simulink library "Lib_EthernetCommunication"  (R2019b)
settings: Solver=VariableStepAuto  StartTime=0.0  StopTime=10.0  RelTol=1e-3
PostLoadFcn:
  | , if any(exist('dsrtsu_mdlpostloadfcn', 'file') == [2, 3, 6]), try dsrtsu_mdlpostloadfcn('Execute', bdroot); catch fprintf('Error in PostLoadFcn (dsrtsu_mdlpostloadfcn) for model "%s":\n %s\n', bdroot, lasterr); end, end,
undefined symbols (not defined in the file): a, acceleration, brake, ddkappa, default_control_command_apollo_bus, default_localization_bus, default_trajectory_bus, dkappa, kappa, n_trajectory_point, relative_time, s, sequence_num, steering_rate, steering_target, theta, throttle, timestamp_sec, v, x, y, z
libraries: rtiethernetudplib x4
settings Model: DSRTSU_INTERNAL_RTI_VER=550  DSRTSU_INTERNAL_RTI_TYPE=rti1401  RTICANMMDATA=struct('GeneralSetupData',struct('modelroot','C:\fav\stack\src\autobox\Simulink\Models','generalsettings',struct('filesettings',struct('destfolder',struct('Name','RTICANMM_FILES','Check',1),'buildfolder',struct('Name','.','Check',1),'AbsDestfolder',struct('Name','C:\fav\stack\src\autobox\Simulink\Models\RTICANMM_FILES'),'AbsBuildfolder',struct('Name','C:\fav\stack\src\autobox\Simulink\Models'))),'options',struct('addpaths',1,'rmpaths',1,'addtrcexclusion',logical(1),'cannavigator',struct('checkmonitoring',0),'show_usrtrc',0,'use_usrtrc',0),'advanced',struct('options',[1 1 1 1 1 1 1 1 1 1 1 1 1 1 1 1 1 1 1 1 1 1 1 1 1 1 1 1 1 1 1 1 1 1 1 1 1 1 1 1 1 1 1 1 1 1 1 1 1 1 1 1 1 1 1 1 1 1 1 1 1 1 1 1 1 1 1 1 1 1 1 1 1 1 1 1 1 1 1 1 1 1 1 1 1 1 1 1 1 1 1 1 1 1 1 1 1 1 1 1]),'MPSetup',{{}},'modelname','Lib_EthernetCommunication','block','Lib_EthernetCommunication'))  DSRTSU_INTERNAL_RTIFPGA=150  Creator=esterle  LastModifiedBy=kessler
settings DataIOCC: ReturnWorkspaceOutputs=off
settings DebuggingCC: ArithmeticOperatorsInVariantConditions=warning
settings SFSimCC: SimUseLocalCustomCode=off  CustomCodeUndefinedFunction=UseInterfaceOnly
settings RTWCC: RTWUseLocalCustomCode=off

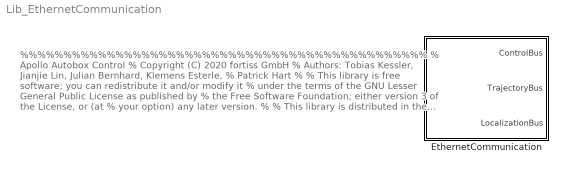
== system Lib_EthernetCommunication ==
  note: %%%%%%%%%%%%%%%%%%%%%%%%%%%%%%%%%%%%%%%%%%%%%%%
      | % Apollo Autobox Control
      | % Copyright (C) 2020 fortiss GmbH
      | % Authors: Tobias Kessler, Jianjie Lin, Julian Bernhard, Klemens Esterle,
      | % Patrick Hart
      | %
      | % This library is free software; you can redistribute it and/or modify it
      | % under the terms of the GNU Lesser General Public License as published by
      | % the Free Software Foundation; either version 3 of the License, or (at
      | % your option) any later version.
      | %
      | % This library is distributed in the hope that it will be useful, but
      | % WITHOUT ANY WARRANTY; without even the implied warranty of
      | % MERCHANTABILITY or FITNESS FOR A PARTICULAR PURPOSE. See the GNU Lesser
      | % General Public License for more details.
      | %
      | % You should have received a copy of the GNU Lesser General Public License
      | % along with this library; if not, write to the Free Software Foundation,
      | % Inc., 51 Franklin Street, Fifth Floor, Boston, MA 02110-1301, USA.
      | %%%%%%%%%%%%%%%%%%%%%%%%%%%%%%%%%%%%%%%%%%%%%%%
  EthernetCommunication : Subsystem

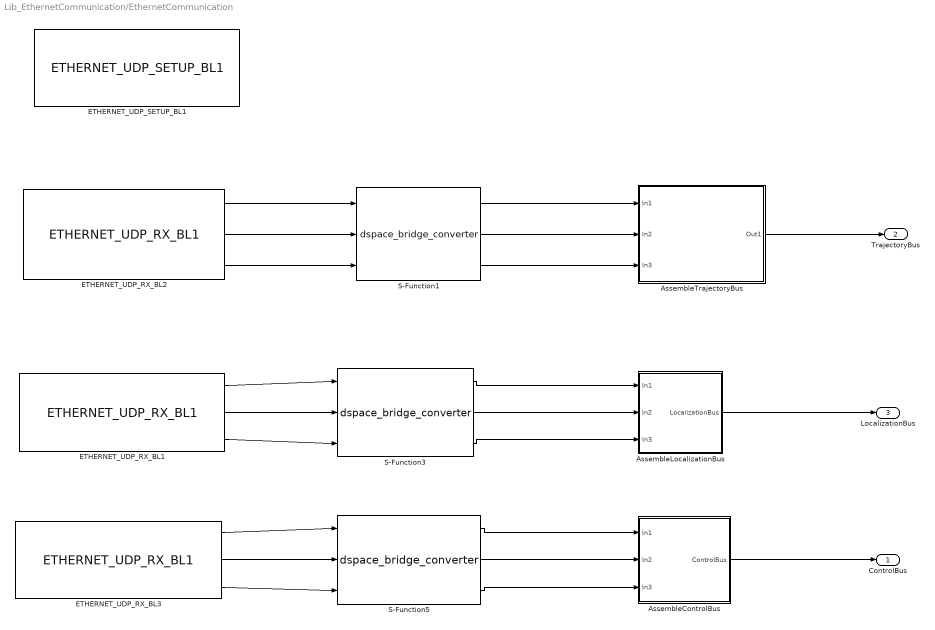
== system Lib_EthernetCommunication/EthernetCommunication ==
  AssembleControlBus : Subsystem
  AssembleLocalizationBus : Subsystem
  AssembleTrajectoryBus : Subsystem
  ETHERNET_UDP_RX_BL1 : rtiethernetudplib/ETHERNET_UDP_RX_BL1  InterfaceName=rti_ethernet_interface_name  BoardType=ETH Type 1  ModuleNo=1  ChannelNo=1  SocketNo=2  MaxMessageSize=1208  LocalSocket=192.168.140.1:5001  RemoteSocket=0.0.0.0:0  DSProperties=struct('RTI',struct('Version',uint32(1),'BlockType',struct('isSLSource',uint8(1),'isSLSink',uint8(0),'isHWSource',uint8(0),'isHWSink',uint8(1),'isSetup',uint8(0),'isInline',uint8(1),'isNonInline',uint8(1),'isInterrupt',uint8(0),'isChannelwise',uint8(1)),'IOBoardType','DSETHERNETUDP','UnitType','ETHUDP','Identifier','RX','DialogType','SL','BlockSet','RTIETHERNETUDP','SlaveProcessor','NONE'))  RTIBlockInterface=struct('OutputPortsWidth',int32([1 1 1]),'OutputPortsActive',[1 1 1],'OutputPortsName',{{'Data',['Message Size'],'Status'}},'OutputPortsDataType',{{'SS_UINT32','SS_INT32','SS_BOOLEAN'}},'BlockDisplay',{{['Ethernet UDP Receive\nBoard Type: ETH Type 1\nModule: 1\nSocket: 2\nMaximum Message Size: 1208'],'center'}},'IconTransparency','on','InitLevel',3,'BlockName',struct('Token',{{'ETHERNET_UDP_RX_BL1'}}),'MaskDescription',['To receive messages from the Ethernet UDP interface.'])  RTIBlockParameters=struct('InterfaceName',{{'rti_ethernet_interface_name','OFF',[]}},'BoardType',{{1,'OFF',[]}},'ModuleNo',{{1,'OFF',[1 16]}},'ChannelNo',{{1,'OFF',[1 2]}},'SocketNo',{{2,'OFF',[1 4]}},'MaxMessageSize',{{1208,'ON',[1 1472]}},'LocalSocket',{{'192.168.140.1:5001','OFF',[]}},'RemoteSocket',{{'0.0.0.0:0','OFF',[]}})  RTISFcnParameters=struct('InterfaceName','char','BoardType','double','ModuleNo','double','ChannelNo','double','SocketNo','double','MaxMessageSize','double','LocalSocket','char','RemoteSocket','char')  RTIBlockParaDefault=struct('InterfaceName','rti_ethernet_interface_name','BoardType',1,'ModuleNo',1,'ChannelNo',1,'SocketNo',1,'MaxMessageSize',625,'LocalSocket','XXX.XXX.XXX.XXX:5000','RemoteSocket','XXX.XXX.XXX.XXX:5000')
      settings: SourceProductName=dSPACE RTI Ethernet (UDP) Blockset
  ETHERNET_UDP_RX_BL2 : rtiethernetudplib/ETHERNET_UDP_RX_BL1  InterfaceName=rti_ethernet_interface_name  BoardType=ETH Type 1  ModuleNo=1  ChannelNo=1  SocketNo=1  MaxMessageSize=1208  LocalSocket=192.168.140.1:5000  RemoteSocket=0.0.0.0:0  DSProperties=struct('RTI',struct('Version',uint32(1),'BlockType',struct('isSLSource',uint8(1),'isSLSink',uint8(0),'isHWSource',uint8(0),'isHWSink',uint8(1),'isSetup',uint8(0),'isInline',uint8(1),'isNonInline',uint8(1),'isInterrupt',uint8(0),'isChannelwise',uint8(1)),'IOBoardType','DSETHERNETUDP','UnitType','ETHUDP','Identifier','RX','DialogType','SL','BlockSet','RTIETHERNETUDP','SlaveProcessor','NONE'))  RTIBlockInterface=struct('OutputPortsWidth',int32([1 1 1]),'OutputPortsActive',[1 1 1],'OutputPortsName',{{'Data',['Message Size'],'Status'}},'OutputPortsDataType',{{'SS_UINT32','SS_INT32','SS_BOOLEAN'}},'BlockDisplay',{{['Ethernet UDP Receive\nBoard Type: ETH Type 1\nModule: 1\nSocket: 1\nMaximum Message Size: 1208'],'center'}},'IconTransparency','on','InitLevel',3,'BlockName',struct('Token',{{'ETHERNET_UDP_RX_BL1'}}),'MaskDescription',['To receive messages from the Ethernet UDP interface.'])  RTIBlockParameters=struct('InterfaceName',{{'rti_ethernet_interface_name','OFF',[]}},'BoardType',{{1,'OFF',[]}},'ModuleNo',{{1,'OFF',[1 16]}},'ChannelNo',{{1,'OFF',[1 2]}},'SocketNo',{{1,'OFF',[1 4]}},'MaxMessageSize',{{1208,'ON',[1 1472]}},'LocalSocket',{{'192.168.140.1:5000','OFF',[]}},'RemoteSocket',{{'0.0.0.0:0','OFF',[]}})  RTISFcnParameters=struct('InterfaceName','char','BoardType','double','ModuleNo','double','ChannelNo','double','SocketNo','double','MaxMessageSize','double','LocalSocket','char','RemoteSocket','char')  RTIBlockParaDefault=struct('InterfaceName','rti_ethernet_interface_name','BoardType',1,'ModuleNo',1,'ChannelNo',1,'SocketNo',1,'MaxMessageSize',625,'LocalSocket','XXX.XXX.XXX.XXX:5000','RemoteSocket','XXX.XXX.XXX.XXX:5000')
      settings: SourceProductName=dSPACE RTI Ethernet (UDP) Blockset
  ETHERNET_UDP_RX_BL3 : rtiethernetudplib/ETHERNET_UDP_RX_BL1  InterfaceName=rti_ethernet_interface_name  BoardType=ETH Type 1  ModuleNo=1  ChannelNo=1  SocketNo=3  MaxMessageSize=1208  LocalSocket=192.168.140.1:5003  RemoteSocket=0.0.0.0:0  DSProperties=struct('RTI',struct('Version',uint32(1),'BlockType',struct('isSLSource',uint8(1),'isSLSink',uint8(0),'isHWSource',uint8(0),'isHWSink',uint8(1),'isSetup',uint8(0),'isInline',uint8(1),'isNonInline',uint8(1),'isInterrupt',uint8(0),'isChannelwise',uint8(1)),'IOBoardType','DSETHERNETUDP','UnitType','ETHUDP','Identifier','RX','DialogType','SL','BlockSet','RTIETHERNETUDP','SlaveProcessor','NONE'))  RTIBlockInterface=struct('OutputPortsWidth',int32([1 1 1]),'OutputPortsActive',[1 1 1],'OutputPortsName',{{'Data',['Message Size'],'Status'}},'OutputPortsDataType',{{'SS_UINT32','SS_INT32','SS_BOOLEAN'}},'BlockDisplay',{{['Ethernet UDP Receive\nBoard Type: ETH Type 1\nModule: 1\nSocket: 3\nMaximum Message Size: 1208'],'center'}},'IconTransparency','on','InitLevel',3,'BlockName',struct('Token',{{'ETHERNET_UDP_RX_BL1'}}),'MaskDescription',['To receive messages from the Ethernet UDP interface.'])  RTIBlockParameters=struct('InterfaceName',{{'rti_ethernet_interface_name','OFF',[]}},'BoardType',{{1,'OFF',[]}},'ModuleNo',{{1,'OFF',[1 16]}},'ChannelNo',{{1,'OFF',[1 2]}},'SocketNo',{{3,'OFF',[1 4]}},'MaxMessageSize',{{1208,'ON',[1 1472]}},'LocalSocket',{{'192.168.140.1:5003','OFF',[]}},'RemoteSocket',{{'0.0.0.0:0','OFF',[]}})  RTISFcnParameters=struct('InterfaceName','char','BoardType','double','ModuleNo','double','ChannelNo','double','SocketNo','double','MaxMessageSize','double','LocalSocket','char','RemoteSocket','char')  RTIBlockParaDefault=struct('InterfaceName','rti_ethernet_interface_name','BoardType',1,'ModuleNo',1,'ChannelNo',1,'SocketNo',1,'MaxMessageSize',625,'LocalSocket','XXX.XXX.XXX.XXX:5000','RemoteSocket','XXX.XXX.XXX.XXX:5000')
      settings: SourceProductName=dSPACE RTI Ethernet (UDP) Blockset
  ETHERNET_UDP_SETUP_BL1 : rtiethernetudplib/ETHERNET_UDP_SETUP_BL1  DSProperties=struct('RTI',struct('Version',uint32(1),'BlockType',struct('isSLSource',uint8(0),'isSLSink',uint8(0),'isHWSource',uint8(0),'isHWSink',uint8(0),'isSetup',uint8(0),'isInline',uint8(1),'isNonInline',uint8(1),'isInterrupt',uint8(0),'isChannelwise',uint8(0)),'IOBoardType','DSETHERNETUDP','UnitType','ETHUDP','Identifier','SETUP','DialogType','ML','BlockSet','RTIETHERNETUDP','SlaveProcessor','NONE'))  RTIBlockInterface=struct('OutputPortsActive',0,'OutputPortsWidth',int32(1),'DialogFcn','rtiethernetudpsetupgui','InitLevel',3,'BlockDisplay',{{['Ethernet UDP Setup\nInterface Name: rti_ethernet_interface_name\nBoard Type: ETH Type 1\nModule: 1\nLocal IP Address: 192.168.140.1'],'center'}},'IconTransparency','on','BlockName',struct('Token',{{'ETHERNET_UDP_SETUP_BL1'}}))  RTIBlockParameters=struct('BoardType',{{1,'OFF',[]}},'ModuleNo',{{1,'ON',[1 16]}},'ChannelNo',{{1,'ON',[1 2]}},'InterfaceName',{{'rti_ethernet_interface_name','OFF',[]}},'LocalIpAddress',{{'192.168.140.1','OFF',[]}},'EnableSocket1',{{1,'OFF',[0 1]}},'LocalPortSocket1',{{'5000','OFF',[0 65535]}},'RemoteIpAddrSocket1',{{'0.0.0.0','OFF',[]}},'RemotePortSocket1',{{'0','OFF',[0 65535]}},'EnableSocket2',{{1,'OFF',[0 1]}},'LocalPortSocket2',{{'5001','OFF',[0 65535]}},'RemoteIpAddrSocket2',{{'0.0.0.0','OFF',[]}},'RemotePortSocket2',{{'0','OFF',[0 65535]}},'EnableSocket3',{{1,'OFF',[0 1]}},'LocalPortSocket3',{{'5003','OFF',[0 65535]}},'RemoteIpAddrSocket3',{{'0.0.0.0','OFF',[]}},'RemotePortSocket3',{{'0','OFF',[0 65535]}},'EnableSocket4',{{0,'OFF',[0 1]}},'LocalPortSocket4',{{'5003','OFF',[0 65535]}},'RemoteIpAddrSocket4',{{'XXX.XXX.XXX.XXX','OFF',[]}},'RemotePortSocket4',{{'5003','OFF',[0 65535]}},'LocalIpAddrHex',{{3232271361,'OFF',[]}},'RemoteIpAddrSocket1Hex',{{0,'OFF',[]}},'RemoteIpAddrSocket2Hex',{{0,'OFF',[]}},'RemoteIpAddrSocket3Hex',{{0,'OFF',[]}},'RemoteIpAddrSocket4Hex',{{0,'OFF',[]}})  RTISFcnParameters=struct('BoardType','double','ModuleNo','double','ChannelNo','double','InterfaceName','char','LocalIpAddress','char','EnableSocket1','double','LocalPortSocket1','double','RemoteIpAddrSocket1','char','RemotePortSocket1','double','EnableSocket2','double','LocalPortSocket2','double','RemoteIpAddrSocket2','char','RemotePortSocket2','double','EnableSocket3','double','LocalPortSocket3','double','RemoteIpAddrSocket3','char','RemotePortSocket3','double','EnableSocket4','double','LocalPortSocket4','double','RemoteIpAddrSocket4','char','RemotePortSocket4','double','LocalIpAddrHex','double','RemoteIpAddrSocket1Hex','double','RemoteIpAddrSocket2Hex','double','RemoteIpAddrSocket3Hex','double','RemoteIpAddrSocket4Hex','double')  RTIBlockParaDefault=struct('BoardType',1,'ModuleNo',1,'ChannelNo',1,'InterfaceName','rti_ethernet_interface_name','LocalIpAddress','XXX.XXX.XXX.XXX','EnableSocket1',0,'LocalPortSocket1',5000,'RemoteIpAddrSocket1','XXX.XXX.XXX.XXX','RemotePortSocket1',5000,'EnableSocket2',0,'LocalPortSocket2',5001,'RemoteIpAddrSocket2','XXX.XXX.XXX.XXX','RemotePortSocket2',5001,'EnableSocket3',0,'LocalPortSocket3',5002,'RemoteIpAddrSocket3','XXX.XXX.XXX.XXX','RemotePortSocket3',5002,'EnableSocket4',0,'LocalPortSocket4',5003,'RemoteIpAddrSocket4','XXX.XXX.XXX.XXX','RemotePortSocket4',5003,'LocalIpAddrHex',0,'RemoteIpAddrSocket1Hex',0,'RemoteIpAddrSocket2Hex',0,'RemoteIpAddrSocket3Hex',0,'RemoteIpAddrSocket4Hex',0)
      settings: SourceProductName=dSPACE RTI Ethernet (UDP) Blockset
  S-Function1 : S-Function  FunctionName=dspace_bridge_converter  SFunctionDeploymentMode=off  EnableBusSupport=off
  S-Function3 : S-Function  FunctionName=dspace_bridge_converter  SFunctionDeploymentMode=off  EnableBusSupport=off
  S-Function5 : S-Function  FunctionName=dspace_bridge_converter  SFunctionDeploymentMode=off  EnableBusSupport=off
  ControlBus : Outport  VectorParamsAs1DForOutWhenUnconnected=off
  "TrajectoryBus " : Outport  Port=2  VectorParamsAs1DForOutWhenUnconnected=off
  "LocalizationBus " : Outport  Port=3  VectorParamsAs1DForOutWhenUnconnected=off
  wires:
  AssembleControlBus/1(ControlBus) -> ControlBus/1
  S-Function5/3 -> AssembleControlBus/3(In3)
  S-Function5/2 -> AssembleControlBus/2(In2)
  S-Function5/1 -> AssembleControlBus/1(In1)
  AssembleLocalizationBus/1("LocalizationBus ") -> "LocalizationBus "/1
  S-Function3/3 -> AssembleLocalizationBus/3(In3)
  S-Function3/2 -> AssembleLocalizationBus/2(In2)
  S-Function3/1 -> AssembleLocalizationBus/1(In1)
  ETHERNET_UDP_RX_BL3/1 -> S-Function5/1
  ETHERNET_UDP_RX_BL3/3 -> S-Function5/3
  ETHERNET_UDP_RX_BL3/2 -> S-Function5/2
  ETHERNET_UDP_RX_BL1/2 -> S-Function3/2
  ETHERNET_UDP_RX_BL1/1 -> S-Function3/1
  ETHERNET_UDP_RX_BL1/3 -> S-Function3/3
  ETHERNET_UDP_RX_BL2/2 -> S-Function1/2
  S-Function1/1 -> AssembleTrajectoryBus/1(In1)
  ETHERNET_UDP_RX_BL2/3 -> S-Function1/3
  ETHERNET_UDP_RX_BL2/1 -> S-Function1/1
  S-Function1/3 -> AssembleTrajectoryBus/3(In3)
  S-Function1/2 -> AssembleTrajectoryBus/2(In2)
  AssembleTrajectoryBus/1(Out1) -> "TrajectoryBus "/1

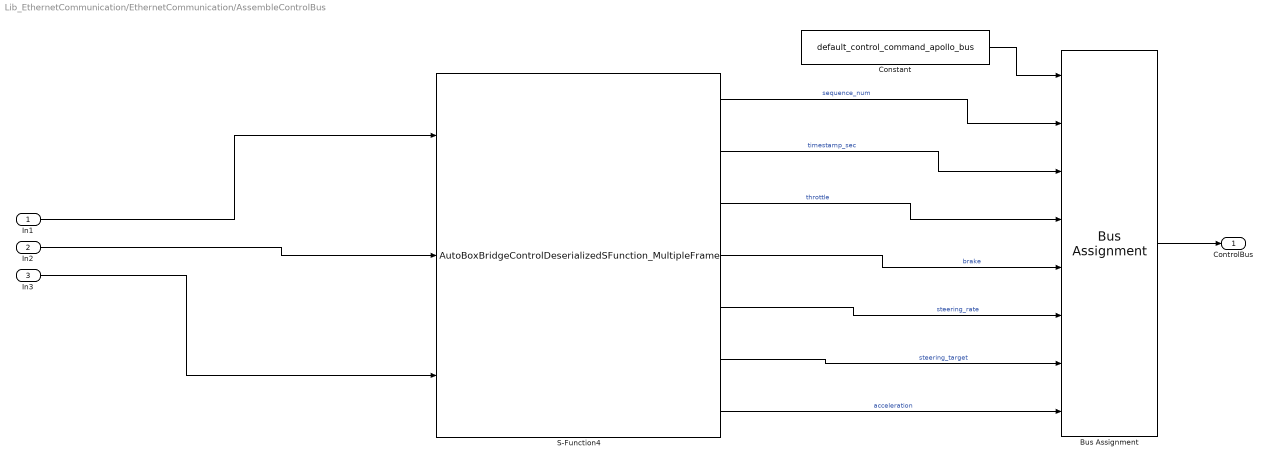
== system Lib_EthernetCommunication/EthernetCommunication/AssembleControlBus ==
  In1 : Inport
  In2 : Inport  Port=2
  In3 : Inport  Port=3
  Bus Assignment : BusAssignment  AssignedSignals=sequence_num,timestamp_sec,throttle,brake,steering_rate,steering_target,acceleration
  Constant : Constant  Value=default_control_command_apollo_bus  OutDataTypeStr=Bus: ControlCommandToAutobox
  S-Function4 : S-Function  FunctionName=AutoBoxBridgeControlDeserializedSFunction_MultipleFrame  SFunctionDeploymentMode=off  EnableBusSupport=off
  ControlBus : Outport  VectorParamsAs1DForOutWhenUnconnected=off
  wires:
  Bus Assignment/1 -> ControlBus/1
  Constant/1 -> Bus Assignment/1
  In2/1 -> S-Function4/2
  In3/1 -> S-Function4/3
  S-Function4/4 -> Bus Assignment/5  "brake"
  S-Function4/7 -> Bus Assignment/8  "acceleration"
  S-Function4/5 -> Bus Assignment/6  "steering_rate"
  S-Function4/3 -> Bus Assignment/4  "throttle"
  S-Function4/1 -> Bus Assignment/2  "sequence_num"
  S-Function4/2 -> Bus Assignment/3  "timestamp_sec"
  In1/1 -> S-Function4/1
  S-Function4/6 -> Bus Assignment/7  "steering_target"

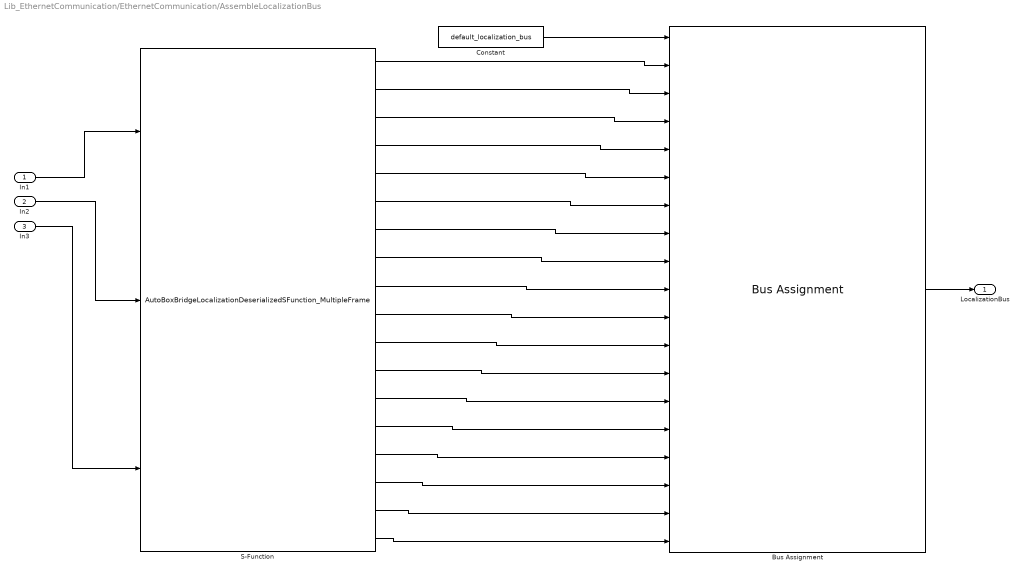
== system Lib_EthernetCommunication/EthernetCommunication/AssembleLocalizationBus ==
  In1 : Inport
  In2 : Inport  Port=2
  In3 : Inport  Port=3
  Bus Assignment : BusAssignment  AssignedSignals=Pose.Orientation.qy,Pose.Orientation.qx,Pose.Orientation.qz,Pose.Orientation.qw,Pose.LinearVelocity.y,Pose.LinearVelocity.x,Pose.LinearVelocity.z,Pose.LinearAcceleration.y,Pose.LinearAcceleration.x,Pose.LinearAcceleration.z,Pose.Position.y,Pose.Position.x,Pose.Position.z,Pose.AngularVelocity.y,Pose.AngularVelocity.x,Pose.AngularVelocity.z,Pose.Heading,MeasurementTime
  Constant : Constant  Value=default_localization_bus  OutDataTypeStr=Bus: LocalizationToAutobox
  S-Function : S-Function  FunctionName=AutoBoxBridgeLocalizationDeserializedSFunction_MultipleFrame  SFunctionDeploymentMode=off  EnableBusSupport=off
  "LocalizationBus " : Outport  VectorParamsAs1DForOutWhenUnconnected=off
  wires:
  In2/1 -> S-Function/2
  S-Function/3 -> Bus Assignment/4
  S-Function/13 -> Bus Assignment/14
  Constant/1 -> Bus Assignment/1
  S-Function/7 -> Bus Assignment/8
  S-Function/5 -> Bus Assignment/6
  S-Function/14 -> Bus Assignment/15
  S-Function/11 -> Bus Assignment/12
  S-Function/15 -> Bus Assignment/16
  In3/1 -> S-Function/3
  S-Function/18 -> Bus Assignment/19
  S-Function/16 -> Bus Assignment/17
  S-Function/12 -> Bus Assignment/13
  S-Function/4 -> Bus Assignment/5
  S-Function/17 -> Bus Assignment/18
  S-Function/8 -> Bus Assignment/9
  S-Function/1 -> Bus Assignment/2
  S-Function/9 -> Bus Assignment/10
  S-Function/2 -> Bus Assignment/3
  S-Function/10 -> Bus Assignment/11
  In1/1 -> S-Function/1
  Bus Assignment/1 -> "LocalizationBus "/1
  S-Function/6 -> Bus Assignment/7

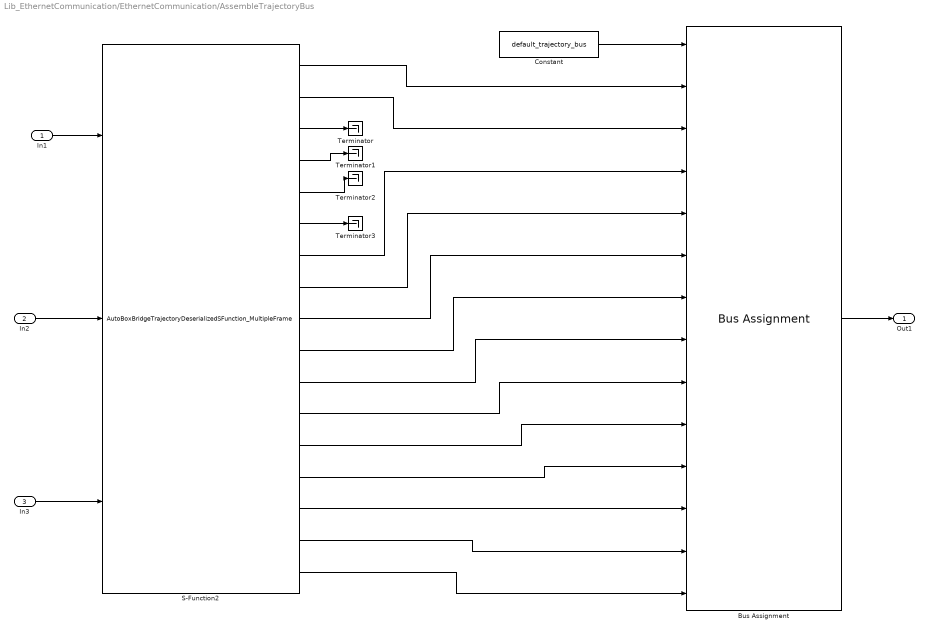
== system Lib_EthernetCommunication/EthernetCommunication/AssembleTrajectoryBus ==
  In1 : Inport
  In2 : Inport  Port=2
  In3 : Inport  Port=3
  Bus Assignment : BusAssignment  AssignedSignals=timestamp_sec,relative_time,x,y,z,a,kappa,theta,dkappa,v,s,n_trajectory_point,ddkappa
  Constant : Constant  Value=default_trajectory_bus  OutDataTypeStr=Bus: ControlTrajectory
  S-Function2 : S-Function  FunctionName=AutoBoxBridgeTrajectoryDeserializedSFunction_MultipleFrame  SFunctionDeploymentMode=off  EnableBusSupport=off
  Terminator{,1..3} (4 alike) : Terminator
  Out1 : Outport
  wires:
  In3/1 -> S-Function2/3
  Bus Assignment/1 -> Out1/1
  S-Function2/14 -> Bus Assignment/11
  In1/1 -> S-Function2/1
  S-Function2/2 -> Bus Assignment/3
  S-Function2/1 -> Bus Assignment/2
  S-Function2/13 -> Bus Assignment/10
  S-Function2/16 -> Bus Assignment/13
  S-Function2/6 -> Terminator3/1
  S-Function2/12 -> Bus Assignment/9
  S-Function2/8 -> Bus Assignment/5
  S-Function2/10 -> Bus Assignment/7
  S-Function2/5 -> Terminator2/1
  S-Function2/17 -> Bus Assignment/14
  S-Function2/11 -> Bus Assignment/8
  S-Function2/9 -> Bus Assignment/6
  S-Function2/7 -> Bus Assignment/4
  In2/1 -> S-Function2/2
  S-Function2/3 -> Terminator/1
  S-Function2/15 -> Bus Assignment/12
  Constant/1 -> Bus Assignment/1
  S-Function2/4 -> Terminator1/1
